simulink model "compare1"  (R2024b)
settings: Solver=VariableStepAuto  StartTime=0.0  StopTime=10.0  RelTol=1e-3
libraries: simulink x9
settings Model: Creator=Ahmad  LastModifiedBy=Ahmad

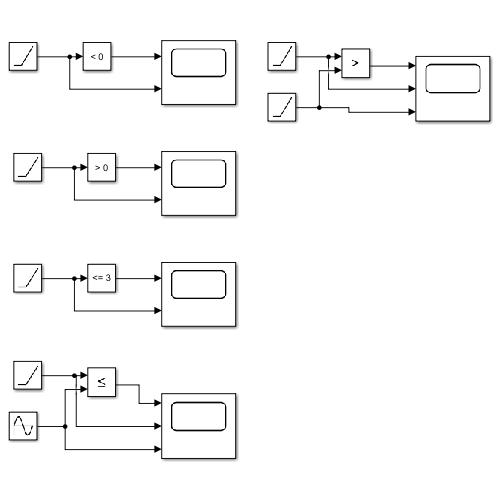
[thumbnail: Simulink's stored preview of the top-level diagram]
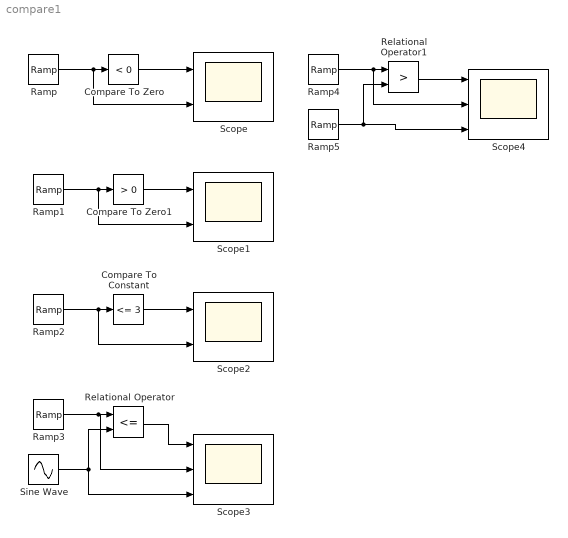
== system compare1 ==
  Compare To Constant : simulink/Logic and Bit Operations/Compare To Constant  relop=<=  const=3  OutDataTypeStr=boolean
  Compare To Zero : simulink/Logic and Bit Operations/Compare To Zero  relop=<  OutDataTypeStr=boolean
  Compare To Zero1 : simulink/Logic and Bit Operations/Compare To Zero  relop=>  OutDataTypeStr=boolean
  Ramp : simulink/Sources/Ramp  slope=-1  start=3  InitialOutput=0
  Ramp{1..4} (4 alike) : simulink/Sources/Ramp  slope=1  start=3  InitialOutput=0
  Ramp5 : simulink/Sources/Ramp  slope=1  start=5  InitialOutput=0
  Relational Operator : RelationalOperator  Operator=<=  OutDataTypeStr=boolean  RndMeth=Simplest  InputSameDT=off
  Relational Operator1 : RelationalOperator  Operator=>  OutDataTypeStr=boolean  RndMeth=Simplest  InputSameDT=off
  Scope : Scope  NumInputPorts=2
  Scope1 : Scope  NumInputPorts=2
  Scope2 : Scope  NumInputPorts=2
  Scope3 : Scope  NumInputPorts=3
  Scope4 : Scope  NumInputPorts=3
  Sine Wave : Sin  SampleTime=0
  wires:
  Ramp/1 -> Scope/2, Compare To Zero/1
  Compare To Zero/1 -> Scope/1
  Compare To Zero1/1 -> Scope1/1
  Ramp1/1 -> Scope1/2, Compare To Zero1/1
  Ramp2/1 -> Scope2/2, Compare To Constant/1
  Compare To Constant/1 -> Scope2/1
  Ramp3/1 -> Scope3/2, Relational Operator/1
  Sine Wave/1 -> Scope3/3, Relational Operator/2
  Relational Operator/1 -> Scope3/1
  Ramp5/1 -> Scope4/3, Relational Operator1/2
  Ramp4/1 -> Scope4/2, Relational Operator1/1
  Relational Operator1/1 -> Scope4/1
